simulink model "Test_Bit_Multiplexer_8_to_1"  (R2023a)
settings: Solver=ode45  StartTime=0.0  StopTime=len  RelTol=1e-3  EnableMultiTasking=on
libraries: simulink x2, Bit_Multiplexers_Lib x1
settings Model: Creator=N  LastModifiedBy=Jozko Mrkvicka
settings SolverCC: AlgebraicLoopSolver=TrustRegion
settings DataIOCC: SaveFormat=Array  ReturnWorkspaceOutputs=off
settings OptimizationCC: LifeSpan=inf
settings DebuggingCC: UnconnectedInputMsg=warning  UnconnectedOutputMsg=warning  UnconnectedLineMsg=warning  SFUnexpectedBacktrackingDiag=warning  SFNoUnconditionalDefaultTransitionDiag=warning  SFExecutionAtInitializationDiag=none  ArithmeticOperatorsInVariantConditions=warning
settings HardwareCC: ProdWordSize=32
settings SFSimCC: SimUseLocalCustomCode=off  CustomCodeUndefinedFunction=UseInterfaceOnly
settings RTWCC: RTWUseLocalCustomCode=off
settings CodeAppCC: StateflowObjectComments=on
settings GRTTargetCC: TargetLangStandard=C89/C90 (ANSI)
settings ConfigComp: CovMetricSettings=dw  CovSaveCumulativeToWorkspaceVar=on  CovSaveSingleToWorkspaceVar=on  CovExternalEMLEnable=off

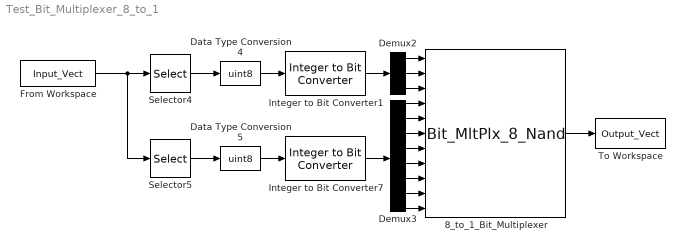
== system Test_Bit_Multiplexer_8_to_1 ==
  8_to_1_Bit_Multiplexer : Bit_Multiplexers_Lib/Bit_MltPlx_8_Nand  SystemSampleTime=-1  VariantActivationTime=update diagram  Latency=0  AutoFrameSizeCalculation=off
  Data Type Conversion4 : DataTypeConversion  OutDataTypeStr=uint8  SaturateOnIntegerOverflow=off  RndMeth=Floor
  Data Type Conversion5 : DataTypeConversion  OutDataTypeStr=uint8  SaturateOnIntegerOverflow=off  RndMeth=Floor
  Demux2 : Demux  Outputs=3
  Demux3 : Demux  Outputs=8
  From Workspace : FromWorkspace  VariableName=Input_Vect  SampleTime=1  Interpolate=off  ZeroCross=off  OutputAfterFinalValue=Holding final value
  Integer to Bit Converter1 : simulink/Logic and Bit Operations/Integer to Bit Converter  nbits=3  signedInputValues=Unsigned  bitOrder=MSB first  outDtype=boolean
      settings: LibrarySourceBlock=|
      | commutil2/Integer to Bit
      | Converter
  Integer to Bit Converter7 : simulink/Logic and Bit Operations/Integer to Bit Converter  nbits=8  signedInputValues=Unsigned  bitOrder=MSB first  outDtype=uint8
      settings: LibrarySourceBlock=|
      | commutil2/Integer to Bit
      | Converter
  Selector4 : Selector  IndexMode=Zero-based  InputPortWidth=2  SampleTime=1  IndexOptions=Index vector (dialog)  Indices=0  OutputSizes=1
  Selector5 : Selector  IndexMode=Zero-based  InputPortWidth=2  IndexOptions=Index vector (dialog)  Indices=1  OutputSizes=1
  To Workspace : ToWorkspace  VariableName=Output_Vect  SampleTime=1
  wires:
  Demux2/1 -> 8_to_1_Bit_Multiplexer/1
  Demux2/2 -> 8_to_1_Bit_Multiplexer/2
  Demux2/3 -> 8_to_1_Bit_Multiplexer/3
  Integer to Bit Converter1/1 -> Demux2/1
  Demux3/1 -> 8_to_1_Bit_Multiplexer/4
  Demux3/2 -> 8_to_1_Bit_Multiplexer/5
  Demux3/3 -> 8_to_1_Bit_Multiplexer/6
  Demux3/4 -> 8_to_1_Bit_Multiplexer/7
  Demux3/5 -> 8_to_1_Bit_Multiplexer/8
  Demux3/6 -> 8_to_1_Bit_Multiplexer/9
  Demux3/7 -> 8_to_1_Bit_Multiplexer/10
  Demux3/8 -> 8_to_1_Bit_Multiplexer/11
  From Workspace/1 -> Selector5/1, Selector4/1
  Selector4/1 -> Data Type Conversion4/1
  Selector5/1 -> Data Type Conversion5/1
  Data Type Conversion4/1 -> Integer to Bit Converter1/1
  Data Type Conversion5/1 -> Integer to Bit Converter7/1
  8_to_1_Bit_Multiplexer/1 -> To Workspace/1
  Integer to Bit Converter7/1 -> Demux3/1
